simulink model "FingerStrokeAssistance"  (R2016a)
settings: Solver=FixedStepDiscrete  StartTime=0.0  StopTime=inf  FixedStep=.001  RelTol=1e-3
PreLoadFcn:
  | settupFilter;
InitFcn:
  | settupFilter;
values from neighbouring files (symbols this model uses):
  x0low = (eye(size(Alow))-Alow)\Blow*0    [settupFilter.m]
undefined symbols (not defined in the file or in its folder): a_hp, Alow, b_hp, Blow, Clow, DiscIntNeverNeededParam, Dlow
libraries: slrtlib x8, simulink x4, xpcnilib x4
settings Model: SimulationMode=external  Creator=Admin  LastModifiedBy=Juno
settings SolverCC: EnableConcurrentExecution=on
settings DataIOCC: LimitDataPoints=on  SaveFormat=Array
settings OptimizationCC: BlockReduction=off  OptimizeBlockIOStorage=off  BufferReuse=off  GlobalBufferReuse=off  ExpressionFolding=off  ExpressionDepthLimit=2147483647  LocalBlockOutputs=off
settings DebuggingCC: UnderspecifiedInitializationDetection=Classic  MergeDetectMultiDrivingBlocksExec=none  SolverPrmCheckMsg=warning  StateNameClashWarn=warning
settings HardwareCC: ProdBitPerPointer=32  ProdLargestAtomicFloat=None  ProdWordSize=32  ProdLongLongMode=on  ProdHWDeviceType=Generic->32-bit x86 compatible
settings ModelReferenceCC: PropagateSignalLabelsOutOfModel=off
settings RTWCC: SystemTargetFile=slrt.tlc  TemplateMakefile=slrt_default_tmf  Description=Simulink Real-Time  RTWCompilerOptimization=on
settings ConfigComp: CovModelRefEnable=Off

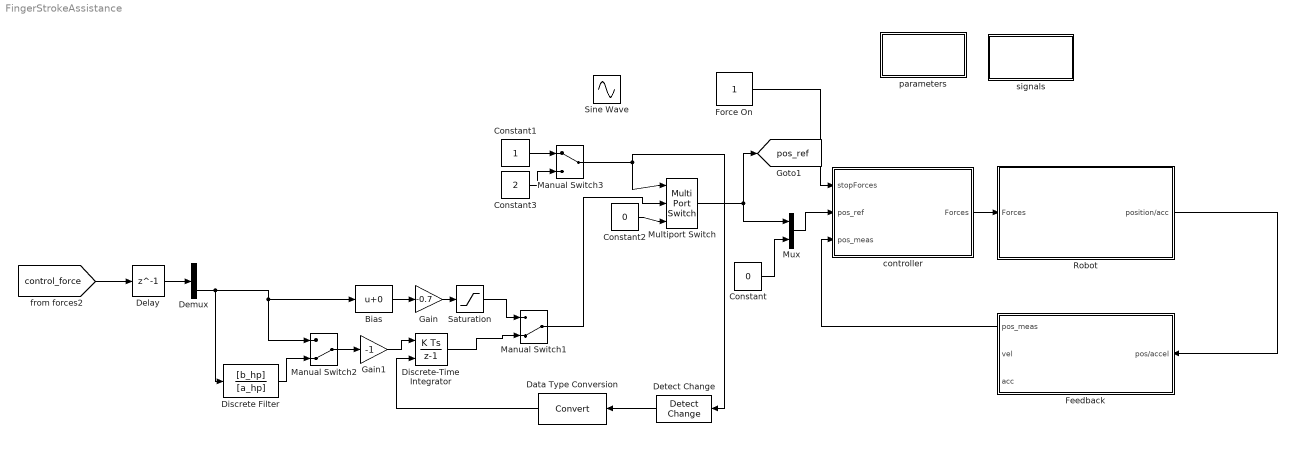
== system FingerStrokeAssistance ==
  Bias : Bias
  Constant : Constant  Value=0
  Constant1 : Constant
  Constant2 : Constant  Value=0
  Constant3 : Constant  Value=2
  Data Type Conversion : DataTypeConversion
  Delay : Delay  DelayLength=1  InitialCondition=0
  Demux : Demux  Outputs=2
  Detect Change : simulink/Logic and Bit Operations/Detect Change  vinit=0  OutDataTypeStr=boolean
  Discrete Filter : DiscreteFilter  Numerator=[b_hp]  Denominator=[a_hp]
  Discrete-Time Integrator : DiscreteIntegrator  ExternalReset=either  InitialCondition=0.1  InitialConditionSetting=State (most efficient)  SampleTime=-1  LimitOutput=on  UpperSaturationLimit=0.9  LowerSaturationLimit=0.1  ICPrevOutput=DiscIntNeverNeededParam  ICPrevScaledInput=DiscIntNeverNeededParam
  Feedback : Subsystem
  Force On : Constant
  Gain : Gain  Gain=-0.7
  Gain1 : Gain  Gain=-1
  Manual Switch1 : ManualSwitch  CurrentSetting=0
  Manual Switch2 : ManualSwitch  CurrentSetting=0
  Manual Switch3 : ManualSwitch
  Multiport Switch : MultiPortSwitch  DataPortOrder=Specify indices  DataPortIndices={1,2}
  Mux : Mux  Inputs=2
  Robot : Subsystem
  Saturation : Saturate  UpperLimit=0.9  LowerLimit=0.1
  Sine Wave : Sin  Amplitude=0.5  Bias=0.5  Frequency=0.5
  controller : Subsystem
  parameters : Subsystem
  signals : Subsystem
  tag scope: pos_ref=global
  wires:
  Robot/1(position/acc) -> Feedback/1(pos/accel)
  controller/1(Forces) -> Robot/1(Forces)
  Force On/1 -> controller/1(stopForces)
  Feedback/1(pos_meas) -> controller/3(pos_meas)
  Constant/1 -> Mux/2
  Mux/1 -> controller/2(pos_ref)
  [control_force] -> Delay/1
  Discrete-Time Integrator/1 -> Manual Switch1/2
  Demux/2 -> Discrete Filter/1, Manual Switch2/1, Bias/1
  Gain/1 -> Saturation/1
  Gain1/1 -> Discrete-Time Integrator/1
  Manual Switch1/1 -> Multiport Switch/2
  Saturation/1 -> Manual Switch1/1
  Delay/1 -> Demux/1
  Bias/1 -> Gain/1
  Manual Switch2/1 -> Gain1/1
  Discrete Filter/1 -> Manual Switch2/2
  Multiport Switch/1 -> Mux/1, [pos_ref]
  Detect Change/1 -> Data Type Conversion/1
  Data Type Conversion/1 -> Discrete-Time Integrator/2
  Constant2/1 -> Multiport Switch/3
  Constant1/1 -> Manual Switch3/1
  Manual Switch3/1 -> Multiport Switch/1, Detect Change/1
  Constant3/1 -> Manual Switch3/2

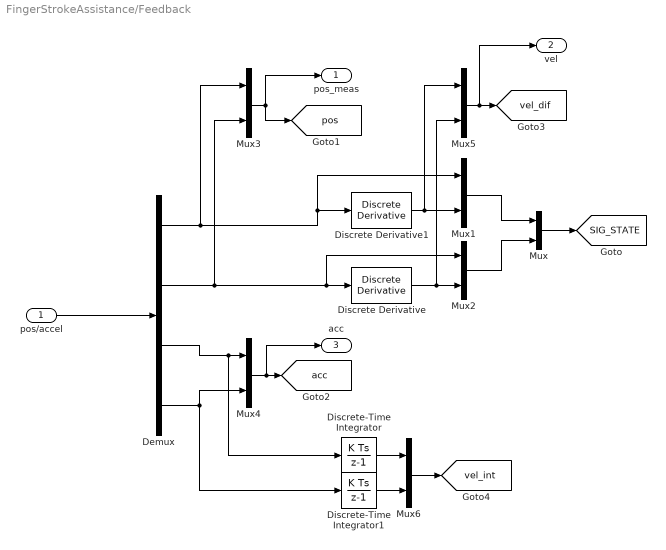
== system FingerStrokeAssistance/Feedback ==
  pos/accel : Inport
  Demux : Demux
  Discrete Derivative : simulink/Discrete/Discrete Derivative  gainval=1.0  ICPrevScaledInput=0.0  InputProcessing=Inherited  OutMin=[]  OutMax=[]  OutDataType=fixdt(1, 16)  OutScaling=2^-10  DoSatur=off
  Discrete Derivative1 : simulink/Discrete/Discrete Derivative  gainval=1.0  ICPrevScaledInput=0.0  InputProcessing=Inherited  OutMin=[]  OutMax=[]  OutDataType=fixdt(1, 16)  OutScaling=2^-10  DoSatur=off
  Discrete-Time Integrator : DiscreteIntegrator  InitialConditionSetting=State (most efficient)  SampleTime=-1  ICPrevOutput=DiscIntNeverNeededParam  ICPrevScaledInput=DiscIntNeverNeededParam
  Discrete-Time Integrator1 : DiscreteIntegrator  InitialConditionSetting=State (most efficient)  SampleTime=-1  ICPrevOutput=DiscIntNeverNeededParam  ICPrevScaledInput=DiscIntNeverNeededParam
  Mux{,1..6} (7 alike) : Mux  Inputs=2
  pos_meas : Outport
  vel : Outport  Port=2
  acc : Outport  Port=3
  tag scope: SIG_STATE=global, acc=global, pos=global, vel_dif=global, vel_int=global
  wires:
  pos/accel/1 -> Demux/1
  Mux/1 -> [SIG_STATE]
  Mux1/1 -> Mux/1
  Mux2/1 -> Mux/2
  Discrete Derivative1/1 -> Mux5/1, Mux1/2
  Discrete Derivative/1 -> Mux5/2, Mux2/2
  Demux/1 -> Mux3/1, Mux1/1, Discrete Derivative1/1
  Demux/2 -> Mux3/2, Mux2/1, Discrete Derivative/1
  Mux3/1 -> pos_meas/1, [pos]
  Demux/3 -> Discrete-Time Integrator/1, Mux4/1
  Demux/4 -> Mux4/2, Discrete-Time Integrator1/1
  Mux4/1 -> acc/1, [acc]
  Mux5/1 -> vel/1, [vel_dif]
  Mux6/1 -> [vel_int]
  Discrete-Time Integrator1/1 -> Mux6/2
  Discrete-Time Integrator/1 -> Mux6/1

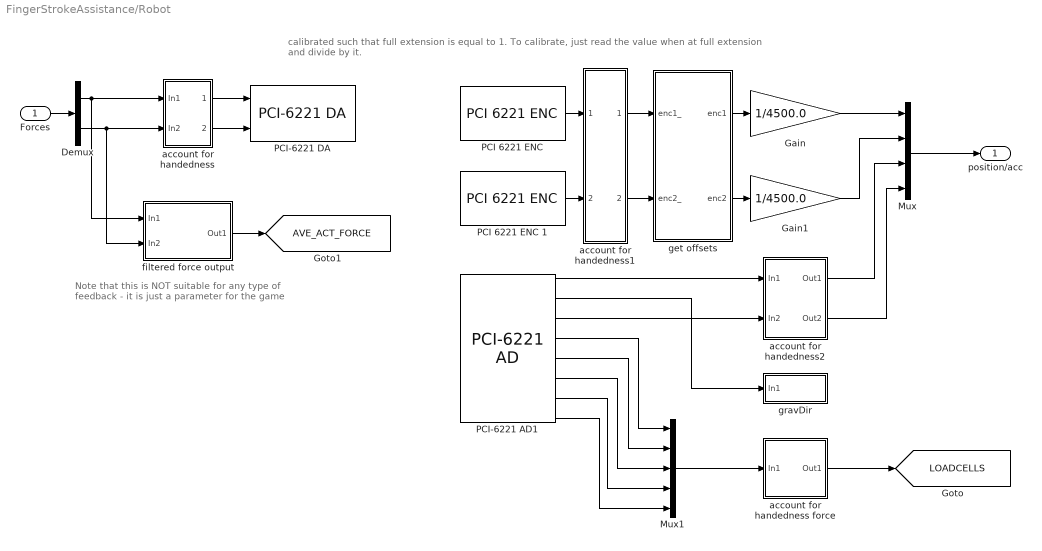
== system FingerStrokeAssistance/Robot ==
  note: Note that this is NOT suitable for any type
      | of feedback - it is just a parameter for the game
  note: calibrated such that full extension is equal to 1. To calibrate, just read the value when at full extension and divide by it.
  Forces : Inport
  Demux : Demux  Outputs=2
  Gain : Gain  Gain=1/4500.0
  Gain1 : Gain  Gain=1/4500.0
  Mux : Mux
  Mux1 : Mux  Inputs=5
  "PCI 6221 ENC " : xpcnilib/Incremental Encoder/PCI 6221 ENC   channel=0  countMode=Quadrature Mode x4  initCount=0  reload=off  indexPhase=A low B low  filter=Minimum pulse width 125 nanoseconds  sampleTime=0.001  slot=-1
  PCI 6221 ENC 1 : xpcnilib/Incremental Encoder/PCI 6221 ENC   channel=1  countMode=Quadrature Mode x4  initCount=0  reload=off  indexPhase=A low B low  filter=Minimum pulse width 125 nanoseconds  sampleTime=0.001  slot=-1
  PCI-6221 AD1 : xpcnilib/A//D/M Series/PCI-6221 AD  channel=[1 2 3 4 5 6 7 8]  range=[10]  coupling=[0]  scantime=5e-6  sampletime=0.001  slot=-1
  PCI-6221 DA : xpcnilib/D//A/M Series/PCI-6221 DA  channel=[1 2]  reset=[1]  initValue=[0]  sampletime=0.001  slot=-1
  account for handedness : Subsystem
  account for handedness force : Subsystem
  account for handedness1 : Subsystem
  account for handedness2 : Subsystem
  filtered force output : Subsystem
  get offsets : Subsystem
  gravDir : Subsystem
  position/acc : Outport
  tag scope: AVE_ACT_FORCE=global, LOADCELLS=global
  wires:
  Gain/1 -> Mux/1
  Mux/1 -> position/acc/1
  Forces/1 -> Demux/1
  Gain1/1 -> Mux/2
  get offsets/1(enc1) -> Gain/1
  get offsets/2(enc2) -> Gain1/1
  Demux/1 -> filtered force output/1(In1), account for handedness/1(In1)
  Demux/2 -> filtered force output/2(In2), account for handedness/2(In2)
  account for handedness/2(Out2) -> PCI-6221 DA/2
  account for handedness/1(Out1) -> PCI-6221 DA/1
  "PCI 6221 ENC "/1 -> account for handedness1/1(In1)
  account for handedness1/1(Out1) -> get offsets/1(enc1_)
  account for handedness1/2(Out2) -> get offsets/2(enc2_)
  PCI 6221 ENC 1/1 -> account for handedness1/2(In2)
  PCI-6221 AD1/1 -> account for handedness2/1(In1)
  PCI-6221 AD1/3 -> account for handedness2/2(In2)
  account for handedness2/1(Out1) -> Mux/3
  account for handedness2/2(Out2) -> Mux/4
  PCI-6221 AD1/4 -> Mux1/1
  PCI-6221 AD1/5 -> Mux1/2
  PCI-6221 AD1/6 -> Mux1/3
  PCI-6221 AD1/7 -> Mux1/4
  PCI-6221 AD1/8 -> Mux1/5
  Mux1/1 -> account for handedness force/1(In1)
  account for handedness force/1(Out1) -> [LOADCELLS]
  PCI-6221 AD1/2 -> gravDir/1(In1)
  filtered force output/1(Out1) -> [AVE_ACT_FORCE]

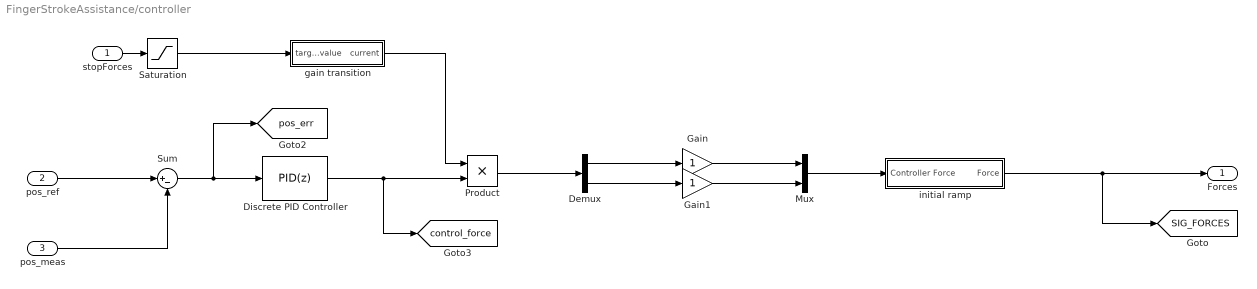
== system FingerStrokeAssistance/controller ==
  stopForces : Inport
  pos_ref : Inport  Port=2
  pos_meas : Inport  Port=3
  Demux : Demux  Outputs=2
  Discrete PID Controller : simulink/Continuous/PID Controller  Controller=PID  TimeDomain=Discrete-time  SampleTime=-1  IntegratorMethod=Forward Euler  FilterMethod=Forward Euler  Form=Parallel  UseFilter=on  ControllerParametersSource=internal  P=10  I=0  D=0.5  N=100  InitialConditionSource=internal  InitialConditionForIntegrator=0  InitialConditionForFilter=0  ExternalReset=none  LimitOutput=off  UpperSaturationLimit=inf  LowerSaturationLimit=-inf  LinearizeAsGain=off  AntiWindupMode=none  Kb=1  TrackingMode=off  Kt=1  PParamMin=[]  PParamMax=[]  IParamMin=[]  IParamMax=[]  DParamMin=[]  DParamMax=[]  NParamMin=[]  NParamMax=[]  KbParamMin=[]  KbParamMax=[]  KtParamMin=[]  KtParamMax=[]  POutMin=[]  POutMax=[]  IOutMin=[]  IOutMax=[]  DOutMin=[]  DOutMax=[]  NOutMin=[]  NOutMax=[]  KbOutMin=[]  KbOutMax=[]  KtOutMin=[]  KtOutMax=[]  IntegratorOutMin=[]  IntegratorOutMax=[]  FilterOutMin=[]  FilterOutMax=[]  SumOutMin=[]  SumOutMax=[]  SumI1OutMin=[]  SumI1OutMax=[]  SumI2OutMin=[]  SumI2OutMax=[]  SumI3OutMin=[]  SumI3OutMax=[]  SumDOutMin=[]  SumDOutMax=[]  SaturationOutMin=[]  SaturationOutMax=[]  IntegratorContinuousStateAttributes=''  IntegratorStateMustResolveToSignalObject=off  IntegratorRTWStateStorageClass=Auto  FilterContinuousStateAttributes=''  FilterStateMustResolveToSignalObject=off  FilterRTWStateStorageClass=Auto  DifferentiatorICPrevScaledInput=0  DifferentiatorOutMin=[]  DifferentiatorOutMax=[]
  Gain : Gain
  Gain1 : Gain
  Mux : Mux  Inputs=2
  Product : Product  RndMeth=Zero
  Saturation : Saturate  UpperLimit=1  LowerLimit=0
  Sum : Sum  Inputs=|+-
  gain transition : Subsystem
  initial ramp : Subsystem
  Forces : Outport
  tag scope: SIG_FORCES=global, control_force=global, pos_err=global
  wires:
  pos_meas/1 -> Sum/2
  stopForces/1 -> Saturation/1
  Saturation/1 -> gain transition/1(target_value)
  Discrete PID Controller/1 -> [control_force], Product/2
  gain transition/1(current) -> Product/1
  initial ramp/1(Force) -> [SIG_FORCES], Forces/1
  Sum/1 -> [pos_err], Discrete PID Controller/1
  pos_ref/1 -> Sum/1
  Product/1 -> Demux/1
  Mux/1 -> initial ramp/1(Controller Force)
  Gain/1 -> Mux/1
  Demux/1 -> Gain/1
  Demux/2 -> Gain1/1
  Gain1/1 -> Mux/2

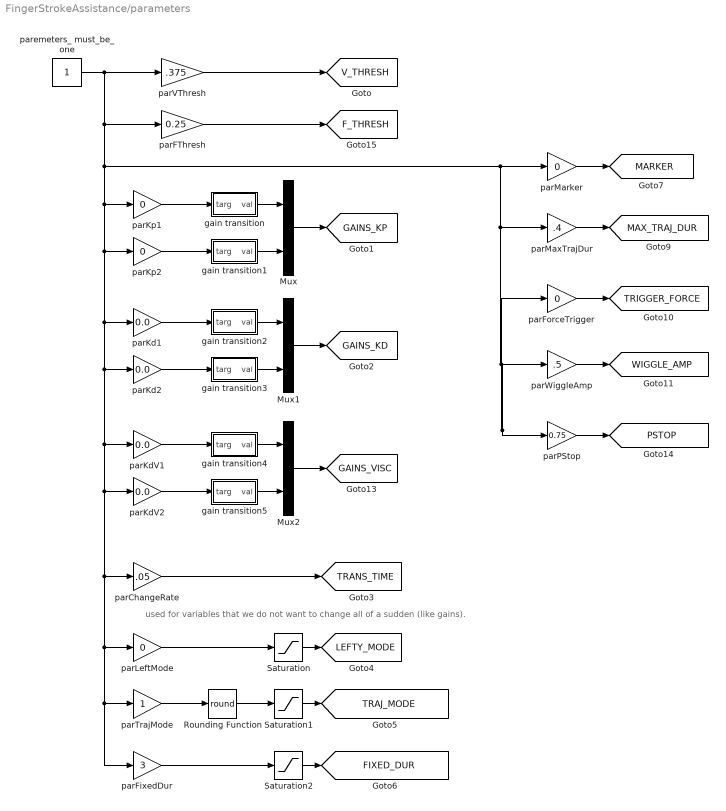
== system FingerStrokeAssistance/parameters ==
  note: used for variables that we do not want to change all of a sudden (like gains).
  Mux : Mux  Inputs=2
  Mux1 : Mux  Inputs=2
  Mux2 : Mux  Inputs=2
  Rounding Function : Rounding  Operator=round
  Saturation : Saturate  UpperLimit=1  LowerLimit=0
  Saturation1 : Saturate  UpperLimit=4  LowerLimit=1
  Saturation2 : Saturate  UpperLimit=10  LowerLimit=.25
  gain transition : Subsystem
  gain transition1 : Subsystem
  gain transition2 : Subsystem
  gain transition3 : Subsystem
  gain transition4 : Subsystem
  gain transition5 : Subsystem
  parChangeRate : Gain  Gain=.05
  parFThresh : Gain  Gain=0.25
  parFixedDur : Gain  Gain=3
  parForceTrigger : Gain  Gain=0
  parKd1 : Gain  Gain=0.0
  parKd2 : Gain  Gain=0.0
  parKdV1 : Gain  Gain=0.0
  parKdV2 : Gain  Gain=0.0
  parKp1 : Gain  Gain=0
  parKp2 : Gain  Gain=0
  parLeftMode : Gain  Gain=0
  parMarker : Gain  Gain=0
  parMaxTrajDur : Gain  Gain=.4
  parPStop : Gain  Gain=0.75
  parTrajMode : Gain
  parVThresh : Gain  Gain=.375
  parWiggleAmp : Gain  Gain=.5
  paremeters_ must_be_one : Constant
  tag scope: FIXED_DUR=global, F_THRESH=global, GAINS_KD=global, GAINS_KP=global, GAINS_VISC=global, LEFTY_MODE=global, MARKER=global, MAX_TRAJ_DUR=global, PSTOP=global, TRAJ_MODE=global, TRANS_TIME=global, TRIGGER_FORCE=global, V_THRESH=global, WIGGLE_AMP=global
  wires:
  Mux/1 -> [GAINS_KP]
  Mux1/1 -> [GAINS_KD]
  Saturation/1 -> [LEFTY_MODE]
  gain transition/1(val) -> Mux/1
  gain transition1/1(val) -> Mux/2
  gain transition2/1(val) -> Mux1/1
  gain transition3/1(val) -> Mux1/2
  parVThresh/1 -> [V_THRESH]
  parKp1/1 -> gain transition/1(targ)
  parKp2/1 -> gain transition1/1(targ)
  parKd1/1 -> gain transition2/1(targ)
  parKd2/1 -> gain transition3/1(targ)
  parChangeRate/1 -> [TRANS_TIME]
  parLeftMode/1 -> Saturation/1
  Saturation1/1 -> [TRAJ_MODE]
  parTrajMode/1 -> Rounding Function/1
  Saturation2/1 -> [FIXED_DUR]
  parFixedDur/1 -> Saturation2/1
  Rounding Function/1 -> Saturation1/1
  parMarker/1 -> [MARKER]
  parMaxTrajDur/1 -> [MAX_TRAJ_DUR]
  parForceTrigger/1 -> [TRIGGER_FORCE]
  parWiggleAmp/1 -> [WIGGLE_AMP]
  Mux2/1 -> [GAINS_VISC]
  gain transition4/1(val) -> Mux2/1
  gain transition5/1(val) -> Mux2/2
  parKdV1/1 -> gain transition4/1(targ)
  parKdV2/1 -> gain transition5/1(targ)
  paremeters_ must_be_one/1 -> parVThresh/1, parFThresh/1, parKp1/1, parKp2/1, parKd1/1, parKd2/1, parKdV1/1, parKdV2/1, parChangeRate/1, parLeftMode/1, parFixedDur/1, parTrajMode/1, parPStop/1, parWiggleAmp/1, parForceTrigger/1, parMaxTrajDur/1, parMarker/1
  parPStop/1 -> [PSTOP]
  parFThresh/1 -> [F_THRESH]

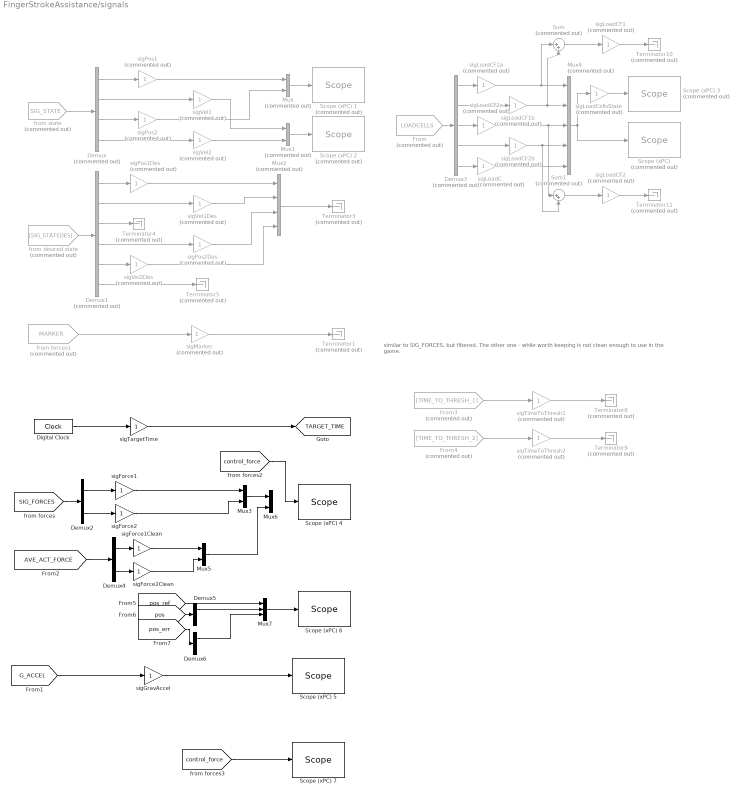
== system FingerStrokeAssistance/signals ==
  note: similar to SIG_FORCES, but filtered. The other one - while worth keeping is not clean enough to use in the game.
  Demux : Demux  Commented=on
  Demux1 : Demux  Commented=on  Outputs=6
  Demux{2,4..6} (4 alike) : Demux  Outputs=2
  Demux3 : Demux  Commented=on  Outputs=5
  Digital Clock : DigitalClock  SampleTime=.001
  From : From  Commented=on  GotoTag=LOADCELLS  TagVisibility=global
  From3 : From  Commented=on  GotoTag=TIME_TO_THRESH_1
  From4 : From  Commented=on  GotoTag=TIME_TO_THRESH_2
  Mux : Mux  Commented=on  Inputs=2
  Mux1 : Mux  Commented=on  Inputs=2
  Mux2 : Mux  Commented=on
  Mux3 : Mux  Inputs=2
  Mux4 : Mux  Commented=on  Inputs=5
  Mux5 : Mux  Inputs=2
  Mux6 : Mux  Inputs=2
  Mux7 : Mux  Inputs=3
  "Scope (xPC) " : slrtlib/Displays and Logging/Scope   Commented=on  scopeno=5  scopetype=Target  autostart=on  viewmode=Graphical redraw  formatstr='%15.6f'  grid=on  ylimits=[-3,3]  nosamples=500  noprepostsamples=0  interleave=1  triggermode=FreeRun  triggersignal=1  trigsignalfromport=off  triggerlevel=0.0  triggerslope=Either  triggerscope=1  triggersample=0  filename=data.dat  mode=Lazy  writesize=512  autorestart=off  dynamicfilemode=off  maxwritefilesize=512*1024^2
  Scope (xPC) 1 : slrtlib/Displays and Logging/Scope   Commented=on  scopeno=1  scopetype=Target  autostart=on  viewmode=Graphical redraw  formatstr='%15.6f'  grid=on  ylimits=[0,1.1]  nosamples=500  noprepostsamples=0  interleave=1  triggermode=FreeRun  triggersignal=1  trigsignalfromport=off  triggerlevel=0.0  triggerslope=Either  triggerscope=1  triggersample=0  filename=data.dat  mode=Lazy  writesize=512  autorestart=off  dynamicfilemode=off  maxwritefilesize=512*1024^2
  Scope (xPC) 2 : slrtlib/Displays and Logging/Scope   Commented=on  scopeno=2  scopetype=Target  autostart=on  viewmode=Graphical redraw  formatstr='%15.6f'  grid=on  ylimits=[-10,10]  nosamples=500  noprepostsamples=0  interleave=1  triggermode=FreeRun  triggersignal=1  trigsignalfromport=off  triggerlevel=0.0  triggerslope=Either  triggerscope=1  triggersample=0  filename=data.dat  mode=Lazy  writesize=512  autorestart=off  dynamicfilemode=off  maxwritefilesize=512*1024^2
  Scope (xPC) 3 : slrtlib/Displays and Logging/Scope   Commented=on  scopeno=4  scopetype=File  autostart=on  viewmode=Graphical redraw  formatstr='%15.6f'  grid=on  ylimits=[0,0]  nosamples=5000  noprepostsamples=0  interleave=1  triggermode=FreeRun  triggersignal=1  trigsignalfromport=off  triggerlevel=0.0  triggerslope=Either  triggerscope=1  triggersample=0  filename=fLogData.dat  mode=Lazy  writesize=512  autorestart=off  dynamicfilemode=off  maxwritefilesize=512*1024^2
  Scope (xPC) 4 : slrtlib/Displays and Logging/Scope   scopeno=1  scopetype=Target  autostart=on  viewmode=Graphical rolling  formatstr='%15.6f'  grid=on  ylimits=[-1,1]  nosamples=2000  noprepostsamples=0  interleave=1  triggermode=FreeRun  triggersignal=1  trigsignalfromport=off  triggerlevel=0.0  triggerslope=Either  triggerscope=1  triggersample=0  filename=data.dat  mode=Lazy  writesize=512  autorestart=off  dynamicfilemode=off  maxwritefilesize=512*1024^2
  Scope (xPC) 5 : slrtlib/Displays and Logging/Scope   scopeno=2  scopetype=Target  autostart=on  viewmode=Graphical rolling  formatstr='%15.6f'  grid=on  ylimits=[-1,1]  nosamples=2000  noprepostsamples=0  interleave=1  triggermode=FreeRun  triggersignal=1  trigsignalfromport=off  triggerlevel=0.0  triggerslope=Either  triggerscope=1  triggersample=0  filename=data.dat  mode=Lazy  writesize=512  autorestart=off  dynamicfilemode=off  maxwritefilesize=512*1024^2
  Scope (xPC) 6 : slrtlib/Displays and Logging/Scope   scopeno=4  scopetype=Target  autostart=on  viewmode=Graphical rolling  formatstr='%15.6f'  grid=on  ylimits=[0,1]  nosamples=2000  noprepostsamples=0  interleave=1  triggermode=FreeRun  triggersignal=1  trigsignalfromport=off  triggerlevel=0.0  triggerslope=Either  triggerscope=1  triggersample=0  filename=data.dat  mode=Lazy  writesize=512  autorestart=off  dynamicfilemode=off  maxwritefilesize=512*1024^2
  Scope (xPC) 7 : slrtlib/Displays and Logging/Scope   scopeno=3  scopetype=Target  autostart=on  viewmode=Numerical  formatstr='%15.6f'  grid=on  ylimits=[.03,.1]  nosamples=10  noprepostsamples=0  interleave=1  triggermode=FreeRun  triggersignal=1  trigsignalfromport=off  triggerlevel=0.0  triggerslope=Either  triggerscope=1  triggersample=0  filename=data.dat  mode=Lazy  writesize=512  autorestart=off  dynamicfilemode=off  maxwritefilesize=512*1024^2
  Sum : Sum  Commented=on  Inputs=|++
  Sum1 : Sum  Commented=on  Inputs=|++
  Terminator{1,3..5,8..11} (8 alike) : Terminator  Commented=on
  from desired state : From  Commented=on  GotoTag=SIG_STATEDES
  from forces1 : From  Commented=on  GotoTag=MARKER  TagVisibility=global
  from state : From  Commented=on  GotoTag=SIG_STATE  TagVisibility=global
  sigForce1 : Gain
  sigForce1Clean : Gain
  sigForce2 : Gain
  sigForce2Clean : Gain
  sigGravAccel : Gain
  sigLoadC : Gain  Commented=on
  sigLoadCF1 : Gain  Commented=on
  sigLoadCF1a : Gain  Commented=on
  sigLoadCF1b : Gain  Commented=on
  sigLoadCF2 : Gain  Commented=on
  sigLoadCF2a : Gain  Commented=on
  sigLoadCF2b : Gain  Commented=on
  sigLoadCellsState : Gain  Commented=on
  sigMarker : Gain  Commented=on
  sigPos1 : Gain  Commented=on
  sigPos1Des : Gain  Commented=on
  sigPos2 : Gain  Commented=on
  sigPos2Des : Gain  Commented=on
  sigTargetTime : Gain
  sigTimeToThresh1 : Gain  Commented=on
  sigTimeToThresh2 : Gain  Commented=on
  sigVel1 : Gain  Commented=on
  sigVel1Des : Gain  Commented=on
  sigVel2 : Gain  Commented=on
  sigVel2Des : Gain  Commented=on
  tag scope: TARGET_TIME=global
  wires:
  from state/1 -> Demux/1
  Demux/1 -> sigPos1/1
  Demux/2 -> sigVel1/1
  Demux/3 -> sigPos2/1
  Demux/4 -> sigVel2/1
  from desired state/1 -> Demux1/1
  Demux1/1 -> sigPos1Des/1
  Demux1/2 -> sigVel1Des/1
  Demux1/3 -> Terminator4/1
  Demux1/4 -> sigPos2Des/1
  Demux1/5 -> sigVel2Des/1
  Demux1/6 -> Terminator5/1
  Mux/1 -> Scope (xPC) 1/1
  Mux1/1 -> Scope (xPC) 2/1
  sigPos1/1 -> Mux/1
  sigPos2/1 -> Mux/2
  sigVel1/1 -> Mux1/1
  sigVel2/1 -> Mux1/2
  sigPos1Des/1 -> Mux2/1
  sigVel1Des/1 -> Mux2/2
  sigPos2Des/1 -> Mux2/3
  sigVel2Des/1 -> Mux2/4
  Mux2/1 -> Terminator3/1
  [SIG_FORCES] -> Demux2/1
  Demux2/1 -> sigForce1/1
  Demux2/2 -> sigForce2/1
  sigForce1/1 -> Mux3/1
  sigForce2/1 -> Mux3/2
  Digital Clock/1 -> sigTargetTime/1
  sigTargetTime/1 -> [TARGET_TIME]
  from forces1/1 -> sigMarker/1
  sigMarker/1 -> Terminator1/1
  From/1 -> Demux3/1
  Demux3/1 -> sigLoadCF1a/1
  Demux3/2 -> sigLoadCF1b/1
  Demux3/3 -> sigLoadCF2a/1
  Demux3/4 -> sigLoadCF2b/1
  Demux3/5 -> sigLoadC/1
  sigLoadCF1a/1 -> Sum/1, Mux4/1
  sigLoadCF1b/1 -> Sum/2, Mux4/2
  sigLoadCF2a/1 -> Sum1/1, Mux4/3
  sigLoadCF2b/1 -> Mux4/4, Sum1/2
  sigLoadC/1 -> Mux4/5
  Mux4/1 -> sigLoadCellsState/1, "Scope (xPC) "/1
  [G_ACCEL] -> sigGravAccel/1
  sigGravAccel/1 -> Scope (xPC) 5/1
  [AVE_ACT_FORCE] -> Demux4/1
  Demux4/1 -> sigForce1Clean/1
  Demux4/2 -> sigForce2Clean/1
  sigForce1Clean/1 -> Mux5/1
  sigForce2Clean/1 -> Mux5/2
  sigTimeToThresh1/1 -> Terminator8/1
  From3/1 -> sigTimeToThresh1/1
  sigTimeToThresh2/1 -> Terminator9/1
  From4/1 -> sigTimeToThresh2/1
  sigLoadCellsState/1 -> Scope (xPC) 3/1
  Sum/1 -> sigLoadCF1/1
  Sum1/1 -> sigLoadCF2/1
  sigLoadCF1/1 -> Terminator10/1
  sigLoadCF2/1 -> Terminator11/1
  Mux3/1 -> Mux6/1
  Mux5/1 -> Mux6/2
  Mux7/1 -> Scope (xPC) 6/1
  [pos_ref] -> Mux7/1
  [control_force] -> Scope (xPC) 4/1
  [pos] -> Demux5/1
  Demux5/1 -> Mux7/2
  [pos_err] -> Demux6/1
  Demux6/1 -> Mux7/3
  [control_force] -> Scope (xPC) 7/1

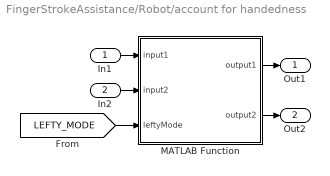
== system FingerStrokeAssistance/Robot/account for handedness ==
  In1 : Inport
  In2 : Inport  Port=2
  MATLAB Function : MATLAB Function  TreatAsAtomicUnit=on
  Out1 : Outport
  Out2 : Outport  Port=2
  wires:
  MATLAB Function/1(output1) -> Out1/1
  MATLAB Function/2(output2) -> Out2/1
  In1/1 -> MATLAB Function/1(input1)
  In2/1 -> MATLAB Function/2(input2)
  [LEFTY_MODE] -> MATLAB Function/3(leftyMode)

== system FingerStrokeAssistance/Robot/account for handedness force ==
  In1 : Inport
  MATLAB Function : MATLAB Function  TreatAsAtomicUnit=on
  Out1 : Outport
  wires:
  [LEFTY_MODE] -> MATLAB Function/2(leftyMode)
  MATLAB Function/1(output) -> Out1/1
  In1/1 -> MATLAB Function/1(inp1)

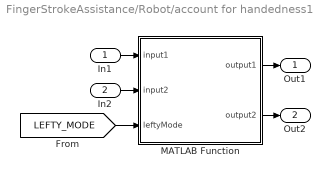
== system FingerStrokeAssistance/Robot/account for handedness1 ==
  In1 : Inport
  In2 : Inport  Port=2
  MATLAB Function : MATLAB Function  TreatAsAtomicUnit=on
  Out1 : Outport
  Out2 : Outport  Port=2
  wires:
  MATLAB Function/1(output1) -> Out1/1
  MATLAB Function/2(output2) -> Out2/1
  In1/1 -> MATLAB Function/1(input1)
  In2/1 -> MATLAB Function/2(input2)
  [LEFTY_MODE] -> MATLAB Function/3(leftyMode)

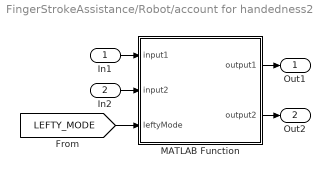
== system FingerStrokeAssistance/Robot/account for handedness2 ==
  In1 : Inport
  In2 : Inport  Port=2
  MATLAB Function : MATLAB Function  TreatAsAtomicUnit=on
  Out1 : Outport
  Out2 : Outport  Port=2
  wires:
  MATLAB Function/1(output1) -> Out1/1
  MATLAB Function/2(output2) -> Out2/1
  In1/1 -> MATLAB Function/1(input1)
  In2/1 -> MATLAB Function/2(input2)
  [LEFTY_MODE] -> MATLAB Function/3(leftyMode)

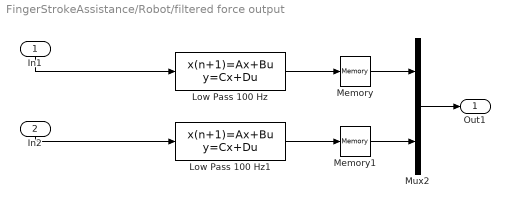
== system FingerStrokeAssistance/Robot/filtered force output ==
  In1 : Inport
  In2 : Inport  Port=2
  Low Pass 100 Hz : DiscreteStateSpace  A=Alow  B=Blow  C=Clow  D=Dlow  X0=x0low  SampleTime=-1
  Low Pass 100 Hz1 : DiscreteStateSpace  A=Alow  B=Blow  C=Clow  D=Dlow  X0=x0low  SampleTime=-1
  Memory : Memory
  Memory1 : Memory
  Mux2 : Mux  Inputs=2
  Out1 : Outport
  wires:
  Low Pass 100 Hz1/1 -> Memory1/1
  Low Pass 100 Hz/1 -> Memory/1
  Mux2/1 -> Out1/1
  In1/1 -> Low Pass 100 Hz/1
  In2/1 -> Low Pass 100 Hz1/1
  Memory/1 -> Mux2/1
  Memory1/1 -> Mux2/2

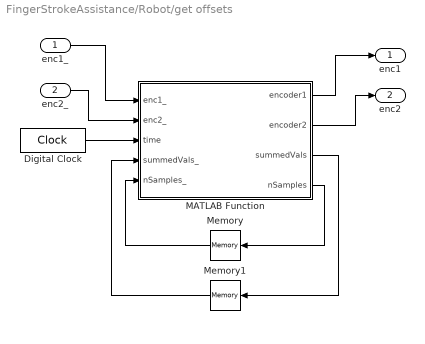
== system FingerStrokeAssistance/Robot/get offsets ==
  enc1_ : Inport
  enc2_ : Inport  Port=2
  Digital Clock : DigitalClock  SampleTime=.001
  MATLAB Function : MATLAB Function  TreatAsAtomicUnit=on
  Memory : Memory
  Memory1 : Memory  X0=[0,0]
  enc1 : Outport
  enc2 : Outport  Port=2
  wires:
  Memory/1 -> MATLAB Function/5(nSamples_)
  Memory1/1 -> MATLAB Function/4(summedVals_)
  MATLAB Function/3(summedVals) -> Memory1/1
  Digital Clock/1 -> MATLAB Function/3(time)
  MATLAB Function/1(encoder1) -> enc1/1
  MATLAB Function/2(encoder2) -> enc2/1
  enc2_/1 -> MATLAB Function/2(enc2_)
  enc1_/1 -> MATLAB Function/1(enc1_)
  MATLAB Function/4(nSamples) -> Memory/1

== system FingerStrokeAssistance/Robot/gravDir ==
  In1 : Inport
  Constant : Constant  Value=1.5
  Sum : Sum  Inputs=|+-
  gain : Gain  Gain=.172
  tag scope: G_ACCEL=global
  wires:
  gain/1 -> [G_ACCEL]
  Sum/1 -> gain/1
  Constant/1 -> Sum/2
  In1/1 -> Sum/1

== system FingerStrokeAssistance/controller/gain transition ==
  target_value : Inport
  Memory : Memory  X0=zeros(1,4)
  gainramp : MATLAB Function  TreatAsAtomicUnit=on
  current : Outport
  wires:
  Memory/1 -> gainramp/3(state)
  gainramp/2(state1) -> Memory/1
  [TRANS_TIME] -> gainramp/1(tr)
  gainramp/1(val) -> current/1
  target_value/1 -> gainramp/2(valD)

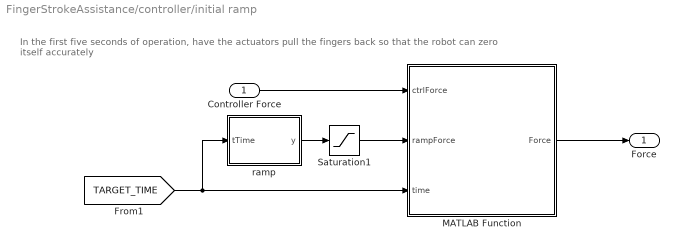
== system FingerStrokeAssistance/controller/initial ramp ==
  note: In the first five seconds of operation, have the actuators pull the fingers back so that the robot can zero itself accurately
  Controller Force : Inport
  MATLAB Function : MATLAB Function  TreatAsAtomicUnit=on
  Saturation1 : Saturate  UpperLimit=2.5  LowerLimit=-2.5
  ramp : MATLAB Function  TreatAsAtomicUnit=on
  Force : Outport
  wires:
  ramp/1(y) -> Saturation1/1
  Controller Force/1 -> MATLAB Function/1(ctrlForce)
  Saturation1/1 -> MATLAB Function/2(rampForce)
  [TARGET_TIME] -> MATLAB Function/3(time), ramp/1(tTime)
  MATLAB Function/1(Force) -> Force/1

== system FingerStrokeAssistance/parameters/gain transition ==
  targ : Inport
  Memory : Memory  X0=zeros(1,4)
  gainramp : MATLAB Function  TreatAsAtomicUnit=on
  val : Outport
  wires:
  Memory/1 -> gainramp/3(state)
  gainramp/2(state1) -> Memory/1
  [TRANS_TIME] -> gainramp/1(tr)
  gainramp/1(val) -> val/1
  targ/1 -> gainramp/2(valD)

== system FingerStrokeAssistance/parameters/gain transition1 ==
  targ : Inport
  Memory : Memory  X0=zeros(1,4)
  gainramp : MATLAB Function  TreatAsAtomicUnit=on
  val : Outport
  wires:
  Memory/1 -> gainramp/3(state)
  gainramp/2(state1) -> Memory/1
  [TRANS_TIME] -> gainramp/1(tr)
  gainramp/1(val) -> val/1
  targ/1 -> gainramp/2(valD)

== system FingerStrokeAssistance/parameters/gain transition2 ==
  targ : Inport
  Memory : Memory  X0=zeros(1,4)
  gainramp : MATLAB Function  TreatAsAtomicUnit=on
  val : Outport
  wires:
  Memory/1 -> gainramp/3(state)
  gainramp/2(state1) -> Memory/1
  [TRANS_TIME] -> gainramp/1(tr)
  gainramp/1(val) -> val/1
  targ/1 -> gainramp/2(valD)

== system FingerStrokeAssistance/parameters/gain transition3 ==
  targ : Inport
  Memory : Memory  X0=zeros(1,4)
  gainramp : MATLAB Function  TreatAsAtomicUnit=on
  val : Outport
  wires:
  Memory/1 -> gainramp/3(state)
  gainramp/2(state1) -> Memory/1
  [TRANS_TIME] -> gainramp/1(tr)
  gainramp/1(val) -> val/1
  targ/1 -> gainramp/2(valD)

== system FingerStrokeAssistance/parameters/gain transition4 ==
  targ : Inport
  Memory : Memory  X0=zeros(1,4)
  gainramp : MATLAB Function  TreatAsAtomicUnit=on
  val : Outport
  wires:
  Memory/1 -> gainramp/3(state)
  gainramp/2(state1) -> Memory/1
  [TRANS_TIME] -> gainramp/1(tr)
  gainramp/1(val) -> val/1
  targ/1 -> gainramp/2(valD)

== system FingerStrokeAssistance/parameters/gain transition5 ==
  targ : Inport
  Memory : Memory  X0=zeros(1,4)
  gainramp : MATLAB Function  TreatAsAtomicUnit=on
  val : Outport
  wires:
  Memory/1 -> gainramp/3(state)
  gainramp/2(state1) -> Memory/1
  [TRANS_TIME] -> gainramp/1(tr)
  gainramp/1(val) -> val/1
  targ/1 -> gainramp/2(valD)

== matlab function FingerStrokeAssistance/controller/gain transition/gainramp ==
  data: val output; tr input; valD input; state1 output; state input
% state contains [valD_,val_,Ro_,t_]
function [val,state1] = fcn(tr,valD,state)
%#eml

% first we need to check if they have changed the desired Value
if ~ (valD == state(1))
    state(1) = valD;
    state(4) = 0;
    state(3) = state(1) - state(2);
end

t = state(4);
Ro = state(3);

if ((t <= tr) && (tr~=0))
    Rd = Ro - Ro*(10*(t)^3/(tr)^3 - 15*(t)^4/(tr)^4 + 6*(t)^5/(tr)^5);
else
    Rd = 0;
end

val = state(1) - Rd;
state(2) = val;
state(4) = t + .001;
state1 = state;

== matlab function FingerStrokeAssistance/Robot/get offsets/MATLAB Function ==
  data: enc1_ input; encoder1 output; enc2_ input; time input; summedVals_ input; nSamples_ input; encoder2 output; summedVals output; nSamples output
%% remove the position offset that comes from using the encoders for
% feedback
%%
function [encoder1, encoder2, summedVals, nSamples] = getOffset(enc1_, enc2_, time, summedVals_, nSamples_)
%#codegen
summedVals = summedVals_;
if (time > 2) && (time < 3)
    summedVals(1) = summedVals_(1) + enc1_;
    summedVals(2) = summedVals_(2) + enc2_;
    nSamples = nSamples_ + 1;
    encoder1 = 0;
    encoder2 = 0;
elseif (time >=3)
    summedVals = summedVals_;
    nSamples = nSamples_;
    encoder1 = enc1_ - summedVals(1)/nSamples;
    encoder2 = enc2_ - summedVals(2)/nSamples;
else (time <= 2)
    summedVals = summedVals_;
    nSamples = nSamples_;
    encoder1 = 0;
    encoder2 = 0;
end

== matlab function FingerStrokeAssistance/controller/initial ramp/MATLAB Function ==
  data: ctrlForce input; Force output; rampForce input; time input
function Force = blendForces(ctrlForce, rampForce, time)
%#codegen
transitionTime = 5.0;
ctrlW = 1 ./ (1 + exp(-8*(time - transitionTime)) );
Force = ctrlW*ctrlForce + (1 - ctrlW)*rampForce;

== matlab function FingerStrokeAssistance/Robot/account for handedness/MATLAB Function ==
  data: input1 input; output1 output; input2 input; leftyMode input; output2 output
% encoder 1 and output 1 relate to the blue mechanism
% encoder 2, output 2 and accel 2 relate to the gold mechanism
% in right hand mode, we want the gold mechanism to control the index finger
% in left hand mode, we want the blue mechanism to control the index finger

% we wallways want the index finger to be finger 1

function [output1, output2] = fcn(input1, input2, leftyMode)
%#codegen
if leftyMode == 1
    output1 = input1;
    output2 = input2;
else
    output1 = input2;
    output2 = input1;
end

== matlab function FingerStrokeAssistance/Robot/account for handedness1/MATLAB Function ==
  data: input1 input; output1 output; input2 input; leftyMode input; output2 output
% encoder 1 and output 1 relate to the blue mechanism
% encoder 2, output 2 and accel 2 relate to the gold mechanism
% in right hand mode, we want the gold mechanism to control the index finger
% in left hand mode, we want the blue mechanism to control the index finger

% we wallways want the index finger to be finger 1

function [output1, output2] = fcn(input1, input2, leftyMode)
%#codegen
if leftyMode == 1
    output1 = input1;
    output2 = input2;
else
    output1 = input2;
    output2 = input1;
end

== matlab function FingerStrokeAssistance/Robot/account for handedness2/MATLAB Function ==
  data: input1 input; output1 output; input2 input; leftyMode input; output2 output
% encoder 1 and output 1 relate to the blue mechanism
% encoder 2, output 2 and accel 2 relate to the gold mechanism
% in right hand mode, we want the gold mechanism to control the index finger
% in left hand mode, we want the blue mechanism to control the index finger

% we wallways want the index finger to be finger 1

function [output1, output2] = fcn(input1, input2, leftyMode)
%#codegen
if leftyMode == 1
    output1 = input1;
    output2 = input2;
else
    output1 = input2;
    output2 = input1;
end

== matlab function FingerStrokeAssistance/parameters/gain transition/gainramp ==
  data: val output; tr input; valD input; state1 output; state input
% state contains [valD_,val_,Ro_,t_]
function [val,state1] = fcn(tr,valD,state)
%#eml

% first we need to check if they have changed the desired Value
if ~ (valD == state(1))
    state(1) = valD;
    state(4) = 0;
    state(3) = state(1) - state(2);
end

t = state(4);
Ro = state(3);

if ((t <= tr) && (tr~=0))
    Rd = Ro - Ro*(10*(t)^3/(tr)^3 - 15*(t)^4/(tr)^4 + 6*(t)^5/(tr)^5);
else
    Rd = 0;
end

val = state(1) - Rd;
state(2) = val;
state(4) = t + .001;
state1 = state;

== matlab function FingerStrokeAssistance/parameters/gain transition1/gainramp ==
  data: val output; tr input; valD input; state1 output; state input
% state contains [valD_,val_,Ro_,t_]
function [val,state1] = fcn(tr,valD,state)
%#eml

% first we need to check if they have changed the desired Value
if ~ (valD == state(1))
    state(1) = valD;
    state(4) = 0;
    state(3) = state(1) - state(2);
end

t = state(4);
Ro = state(3);

if ((t <= tr) && (tr~=0))
    Rd = Ro - Ro*(10*(t)^3/(tr)^3 - 15*(t)^4/(tr)^4 + 6*(t)^5/(tr)^5);
else
    Rd = 0;
end

val = state(1) - Rd;
state(2) = val;
state(4) = t + .001;
state1 = state;

== matlab function FingerStrokeAssistance/parameters/gain transition2/gainramp ==
  data: val output; tr input; valD input; state1 output; state input
% state contains [valD_,val_,Ro_,t_]
function [val,state1] = fcn(tr,valD,state)
%#eml

% first we need to check if they have changed the desired Value
if ~ (valD == state(1))
    state(1) = valD;
    state(4) = 0;
    state(3) = state(1) - state(2);
end

t = state(4);
Ro = state(3);

if ((t <= tr) && (tr~=0))
    Rd = Ro - Ro*(10*(t)^3/(tr)^3 - 15*(t)^4/(tr)^4 + 6*(t)^5/(tr)^5);
else
    Rd = 0;
end

val = state(1) - Rd;
state(2) = val;
state(4) = t + .001;
state1 = state;

== matlab function FingerStrokeAssistance/parameters/gain transition3/gainramp ==
  data: val output; tr input; valD input; state1 output; state input
% state contains [valD_,val_,Ro_,t_]
function [val,state1] = fcn(tr,valD,state)
%#eml

% first we need to check if they have changed the desired Value
if ~ (valD == state(1))
    state(1) = valD;
    state(4) = 0;
    state(3) = state(1) - state(2);
end

t = state(4);
Ro = state(3);

if ((t <= tr) && (tr~=0))
    Rd = Ro - Ro*(10*(t)^3/(tr)^3 - 15*(t)^4/(tr)^4 + 6*(t)^5/(tr)^5);
else
    Rd = 0;
end

val = state(1) - Rd;
state(2) = val;
state(4) = t + .001;
state1 = state;

== matlab function FingerStrokeAssistance/Robot/account for handedness force/MATLAB Function ==
  data: inp1 input; output output; leftyMode input
% channel1 - gold tip
% channel2 - blue tip
% channel3 - gold base
% channel4 - blue base
% we wallways want the index finger to be finger 1

function output = fcn(inp1, leftyMode)
%#codegen

if leftyMode == 1
    output = [inp1(4); inp1(2); inp1(3); inp1(1); inp1(5)];
else
    output = [inp1(3); inp1(1); inp1(4); inp1(2); inp1(5)];
    %output = [inp1(3,1); inp1(4,2); inp1(5)];
end

== matlab function FingerStrokeAssistance/parameters/gain transition4/gainramp ==
  data: val output; tr input; valD input; state1 output; state input
% state contains [valD_,val_,Ro_,t_]
function [val,state1] = fcn(tr,valD,state)
%#eml

% first we need to check if they have changed the desired Value
if ~ (valD == state(1))
    state(1) = valD;
    state(4) = 0;
    state(3) = state(1) - state(2);
end

t = state(4);
Ro = state(3);

if ((t <= tr) && (tr~=0))
    Rd = Ro - Ro*(10*(t)^3/(tr)^3 - 15*(t)^4/(tr)^4 + 6*(t)^5/(tr)^5);
else
    Rd = 0;
end

val = state(1) - Rd;
state(2) = val;
state(4) = t + .001;
state1 = state;

== matlab function FingerStrokeAssistance/parameters/gain transition5/gainramp ==
  data: val output; tr input; valD input; state1 output; state input
% state contains [valD_,val_,Ro_,t_]
function [val,state1] = fcn(tr,valD,state)
%#eml

% first we need to check if they have changed the desired Value
if ~ (valD == state(1))
    state(1) = valD;
    state(4) = 0;
    state(3) = state(1) - state(2);
end

t = state(4);
Ro = state(3);

if ((t <= tr) && (tr~=0))
    Rd = Ro - Ro*(10*(t)^3/(tr)^3 - 15*(t)^4/(tr)^4 + 6*(t)^5/(tr)^5);
else
    Rd = 0;
end

val = state(1) - Rd;
state(2) = val;
state(4) = t + .001;
state1 = state;

== matlab function FingerStrokeAssistance/controller/initial ramp/ramp ==
  data: tTime input; y output
function y = fcn(tTime)
%#codegen
slope = -0.8;
y = tTime*slope;
